simulink model "hbridge_lcl_grid_following"  (R2025b)
settings: Solver=FixedStepDiscrete  StartTime=0.0  StopTime=T_sim_gfl  FixedStep=T_step_grid  RelTol=1e-3
values from neighbouring files (symbols this model uses):
  P_ref_final = 500.0    (= 500)    [grid_following_params.m]
  Q_ref_test = 150.0    (= 150)    [grid_following_params.m]
  T_control_gfl = 1/f_sw_grid    [grid_following_params.m]
  t_power_ramp = 0.10    (= 0.1)    [grid_following_params.m]
  t_q_step = 0.32    [grid_following_params.m]
  V_grid_pk = sqrt(2)*V_grid_rms    [grid_tie_params.m]
  Vdc_grid = 48.0    (= 48)    [grid_tie_params.m]
  w_grid_tie = 2*pi*f_grid_tie    (= 314.159265359)    [grid_tie_params.m]
libraries: simulink x3
settings Model: Creator=hemanggadhvi  LastModifiedBy=hemanggadhvi

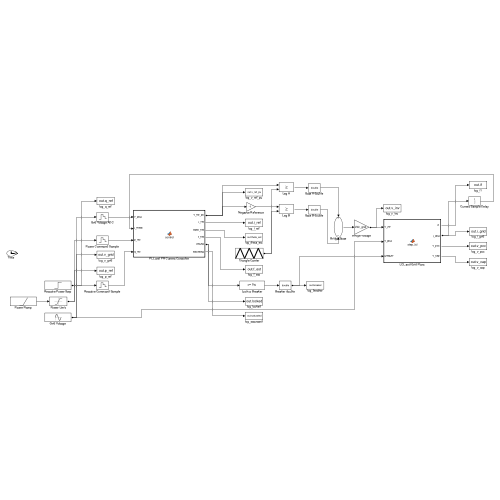
[thumbnail: Simulink's stored preview of the top-level diagram]
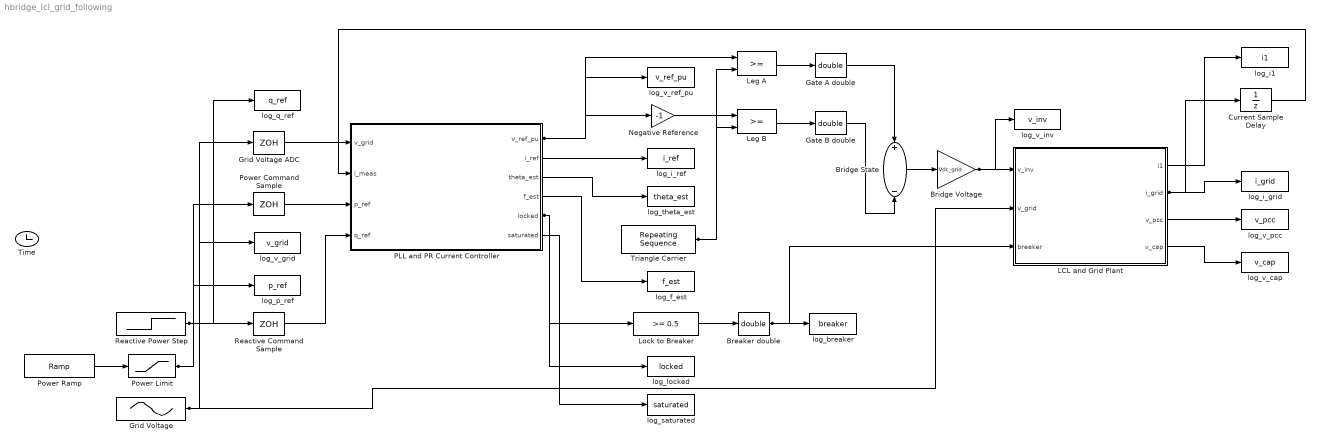
== system hbridge_lcl_grid_following ==
  Breaker double : DataTypeConversion  OutDataTypeStr=double  SaturateOnIntegerOverflow=off  RndMeth=Floor
  Bridge State : Sum  Inputs=+-
  Bridge Voltage : Gain  Gain=Vdc_grid
  Current Sample Delay : UnitDelay  SampleTime=T_control_gfl  HasFrameUpgradeWarning=on
  Gate A double : DataTypeConversion  OutDataTypeStr=double  SaturateOnIntegerOverflow=off  RndMeth=Floor
  Gate B double : DataTypeConversion  OutDataTypeStr=double  SaturateOnIntegerOverflow=off  RndMeth=Floor
  Grid Voltage : Sin  Amplitude=V_grid_pk  Frequency=w_grid_tie  SampleTime=0
  Grid Voltage ADC : ZeroOrderHold  SampleTime=T_control_gfl
  LCL and Grid Plant : MATLAB Function  TreatAsAtomicUnit=on
  Leg A : RelationalOperator  OutDataTypeStr=boolean  RndMeth=Simplest  InputSameDT=off
  Leg B : RelationalOperator  OutDataTypeStr=boolean  RndMeth=Simplest  InputSameDT=off
  Lock to Breaker : simulink/Logic and Bit Operations/Compare To Constant  relop=>=  const=0.5  OutDataTypeStr=boolean
  Negative Reference : Gain  Gain=-1
  PLL and PR Current Controller : MATLAB Function  TreatAsAtomicUnit=on
  Power Command Sample : ZeroOrderHold  SampleTime=T_control_gfl
  Power Limit : Saturate  UpperLimit=P_ref_final  LowerLimit=0
  Power Ramp : simulink/Sources/Ramp  slope=P_ref_final/t_power_ramp  start=t_power_start  InitialOutput=0
  Reactive Command Sample : ZeroOrderHold  SampleTime=T_control_gfl
  Reactive Power Step : Step  Time=t_q_step  After=Q_ref_test  SampleTime=0
  Time : Clock
  Triangle Carrier : simulink/Sources/Repeating Sequence  rep_seq_t=carrier_time_grid  rep_seq_y=carrier_values_grid
  log_breaker : ToWorkspace  VariableName=breaker  SaveFormat=Timeseries  SampleTime=-1
  log_f_est : ToWorkspace  VariableName=f_est  SaveFormat=Timeseries  SampleTime=-1
  log_i1 : ToWorkspace  VariableName=i1  SaveFormat=Timeseries  SampleTime=-1
  log_i_grid : ToWorkspace  VariableName=i_grid  SaveFormat=Timeseries  SampleTime=-1
  log_i_ref : ToWorkspace  VariableName=i_ref  SaveFormat=Timeseries  SampleTime=-1
  log_locked : ToWorkspace  VariableName=locked  SaveFormat=Timeseries  SampleTime=-1
  log_p_ref : ToWorkspace  VariableName=p_ref  SaveFormat=Timeseries  SampleTime=-1
  log_q_ref : ToWorkspace  VariableName=q_ref  SaveFormat=Timeseries  SampleTime=-1
  log_saturated : ToWorkspace  VariableName=saturated  SaveFormat=Timeseries  SampleTime=-1
  log_theta_est : ToWorkspace  VariableName=theta_est  SaveFormat=Timeseries  SampleTime=-1
  log_v_cap : ToWorkspace  VariableName=v_cap  SaveFormat=Timeseries  SampleTime=-1
  log_v_grid : ToWorkspace  VariableName=v_grid  SaveFormat=Timeseries  SampleTime=-1
  log_v_inv : ToWorkspace  VariableName=v_inv  SaveFormat=Timeseries  SampleTime=-1
  log_v_pcc : ToWorkspace  VariableName=v_pcc  SaveFormat=Timeseries  SampleTime=-1
  log_v_ref_pu : ToWorkspace  VariableName=v_ref_pu  SaveFormat=Timeseries  SampleTime=-1
  wires:
  Current Sample Delay/1 -> PLL and PR Current Controller/2(i_meas)
  LCL and Grid Plant/3(v_pcc) -> log_v_pcc/1
  LCL and Grid Plant/1(i1) -> log_i1/1
  Bridge Voltage/1 -> log_v_inv/1, LCL and Grid Plant/1(v_inv)
  Bridge State/1 -> Bridge Voltage/1
  Gate B double/1 -> Bridge State/2
  Gate A double/1 -> Bridge State/1
  Lock to Breaker/1 -> Breaker double/1
  PLL and PR Current Controller/3(theta_est) -> log_theta_est/1
  Triangle Carrier/1 -> Leg B/2, Leg A/2
  LCL and Grid Plant/4(v_cap) -> log_v_cap/1
  Leg A/1 -> Gate A double/1
  PLL and PR Current Controller/6(saturated) -> log_saturated/1
  Negative Reference/1 -> Leg B/1
  PLL and PR Current Controller/5(locked) -> log_locked/1, Lock to Breaker/1
  PLL and PR Current Controller/4(f_est) -> log_f_est/1
  Reactive Power Step/1 -> log_q_ref/1, Reactive Command Sample/1
  Power Command Sample/1 -> PLL and PR Current Controller/3(p_ref)
  PLL and PR Current Controller/2(i_ref) -> log_i_ref/1
  Breaker double/1 -> log_breaker/1, LCL and Grid Plant/3(breaker)
  Leg B/1 -> Gate B double/1
  PLL and PR Current Controller/1(v_ref_pu) -> log_v_ref_pu/1, Negative Reference/1, Leg A/1
  LCL and Grid Plant/2(i_grid) -> log_i_grid/1, Current Sample Delay/1
  Reactive Command Sample/1 -> PLL and PR Current Controller/4(q_ref)
  Power Ramp/1 -> Power Limit/1
  Grid Voltage ADC/1 -> PLL and PR Current Controller/1(v_grid)
  Grid Voltage/1 -> log_v_grid/1, Grid Voltage ADC/1, LCL and Grid Plant/2(v_grid)
  Power Limit/1 -> log_p_ref/1, Power Command Sample/1

== matlab function hbridge_lcl_grid_following/LCL and Grid Plant ==
  data: v_inv input; i1 output; v_grid input; breaker input; i_grid output; v_pcc output; v_cap output
function [i1,i_grid,v_pcc,v_cap] = step_lcl(v_inv,v_grid,breaker)
%#codegen
persistent x_i1 x_ig x_vc
if isempty(x_i1); x_i1=0; x_ig=0; x_vc=0; end
Ts=9.9999999999999995e-07; L1=0.00014999999999999999; R1=0.014999999999999999; C=2.0000000000000002e-05; Rd=0.56000000000000005; L2=9.4999999999999992e-05; R2=0.065000000000000002;
if breaker<0.5; x_ig=0; end; ic=x_i1-x_ig; vn=x_vc+Rd*ic;
di1=(v_inv-R1*x_i1-vn)/L1; dvc=ic/C;
if breaker>=0.5; dig=(vn-R2*x_ig-v_grid)/L2; else; dig=0; end
x_i1=x_i1+Ts*di1; x_vc=x_vc+Ts*dvc;
if breaker>=0.5; x_ig=x_ig+Ts*dig; else; x_ig=0; end
i1=x_i1; i_grid=x_ig; v_cap=x_vc; v_pcc=x_vc+Rd*(x_i1-x_ig);
end

== matlab function hbridge_lcl_grid_following/PLL and PR Current Controller ==
  data: v_grid input; v_ref_pu output; i_meas input; p_ref input; q_ref input; i_ref output; theta_est output; f_est output; locked output; saturated output
function [v_ref_pu,i_ref,theta_est,f_est,locked,saturated] = control(v_grid,i_meas,p_ref,q_ref)
%#codegen
persistent va vb theta omega pll_i lock_count xr1 xr2 iref_old
if isempty(va); va=0; vb=0; theta=0; omega=2*pi*50; pll_i=0; lock_count=0; xr1=0; xr2=0; iref_old=0; end
Ts=5.0000000000000002e-05; Vpk=40.799999999999997; Vrms=28.849956672411135; Vdc=48;
% SOGI and normalized SRF PLL, Heun state update
dva1=1.4142135623730951*omega*(v_grid-va)-omega*vb; dvb1=omega*va;
va_p=va+Ts*dva1; vb_p=vb+Ts*dvb1;
dva2=1.4142135623730951*omega*(v_grid-va_p)-omega*vb_p; dvb2=omega*va_p;
va=va+0.5*Ts*(dva1+dva2); vb=vb+0.5*Ts*(dvb1+dvb2);
amp=sqrt(va*va+vb*vb); q=(va*cos(theta)+vb*sin(theta))/max(amp,0.1*Vpk);
unsat_w=2*pi*50+106.61308829222321*q+pll_i; wmin=2*pi*45; wmax=2*pi*55; omega=min(max(unsat_w,wmin),wmax);
if (unsat_w==omega)||(unsat_w>wmax&&q<0)||(unsat_w<wmin&&q>0); pll_i=pll_i+Ts*5684.8921350274704*q; end
theta=mod(theta+Ts*omega,2*pi);
if amp>0.7*Vpk && abs(q)<0.040000000000000001 && abs(omega/(2*pi)-50)<0.2; lock_count=min(lock_count+1,200); else; lock_count=0; end
locked=double(lock_count>=200);
% Active/reactive current command and grid-voltage feedforward
theta_current=theta-2.5*omega*Ts;
i_ref=locked*(sqrt(2)/Vrms)*(p_ref*sin(theta_current)-q_ref*cos(theta_current)); di_ref=(i_ref-iref_old)/Ts; iref_old=i_ref;
err=i_ref-i_meas; resonant=2*31.415926535897931*xr2;
v_ff=v_grid+0.065000000000000002*i_ref+0.00024499999999999999*di_ref; v_ctrl=0.65000000000000002*err+28*resonant;
v_unsat=v_ff+v_ctrl; vmax=0.94999999999999996*Vdc; v_cmd=min(max(v_unsat,-vmax),vmax); saturated=double(v_cmd~=v_unsat);
% Band-limited resonant state; freeze when saturation would increase error
if ~saturated || sign(err)~=sign(v_unsat-v_cmd);
 dx1=xr2; dx2=err-(2*31.415926535897931)*xr2-(2*pi*50)^2*xr1;
 x1p=xr1+Ts*dx1; x2p=xr2+Ts*dx2;
 dx1p=x2p; dx2p=err-(2*31.415926535897931)*x2p-(2*pi*50)^2*x1p;
 xr1=xr1+0.5*Ts*(dx1+dx1p); xr2=xr2+0.5*Ts*(dx2+dx2p); end
v_ref_pu=v_cmd/Vdc; theta_est=theta; f_est=omega/(2*pi);
end
